simulink model "MinTimeClimbSim"  (R2019a)
settings: Solver=ode1  StartTime=0.0  StopTime=600  FixedStep=tstep  RelTol=1e-3
InitFcn:
  | initSim;
StopFcn:
  | plotSimSolution;
values from neighbouring files (symbols this model uses):
  par = problem.data    [initSim.m]
  tstep = 0.1    [initSim.m]
undefined symbols (not defined in the file or in its folder): F, m, MIL, Moderate, problem
libraries: aerolibwind2 x1, sharedtransform x1
settings Model: Creator=yn15  LastModifiedBy=Yuanb
settings DataIOCC: ReturnWorkspaceOutputs=off
settings OptimizationCC: LifeSpan=inf
settings DebuggingCC: SFUnexpectedBacktrackingDiag=warning  SFNoUnconditionalDefaultTransitionDiag=warning  SFExecutionAtInitializationDiag=none  ArithmeticOperatorsInVariantConditions=warning
settings SFSimCC: SimUseLocalCustomCode=off
settings RTWCC: RTWUseLocalCustomCode=off
settings CodeAppCC: StateflowObjectComments=on
settings GRTTargetCC: TargetLangStandard=C89/C90 (ANSI)
settings ConfigComp: CovMetricSettings=dw  CovHtmlReporting=on  CovSaveCumulativeToWorkspaceVar=on  CovSaveSingleToWorkspaceVar=on  CovExternalEMLEnable=off

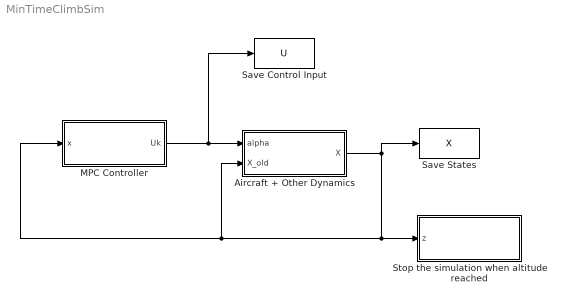
== system MinTimeClimbSim ==
  Aircraft + Other Dynamics : Subsystem
  "MPC Controller " : Subsystem
  Save Control Input : ToWorkspace  VariableName=U  SampleTime=-1
      settings: Save2DSignal=2-D array (concatenate along first dimension)
  Save States : ToWorkspace  VariableName=X  SampleTime=-1
  "Stop the simulation when altitude reached " : Subsystem
  wires:
  "MPC Controller "/1(Uk) -> Aircraft + Other Dynamics/1(alpha), Save Control Input/1
  Aircraft + Other Dynamics/1(X) -> Save States/1, "Stop the simulation when altitude reached "/1(z), Aircraft + Other Dynamics/2("X_old "), "MPC Controller "/1(x)

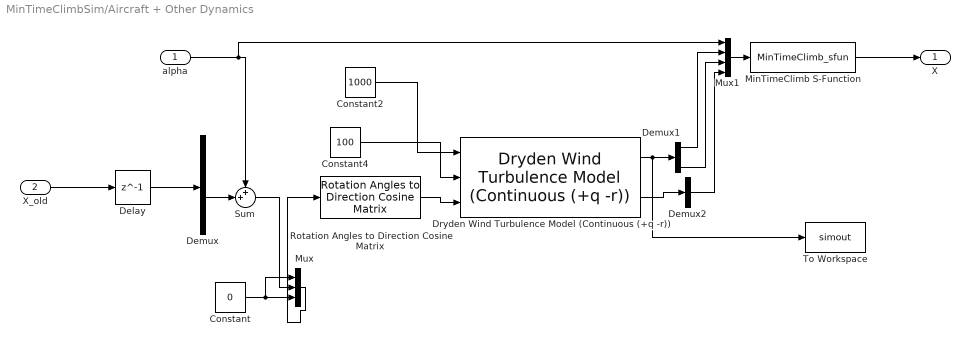
== system MinTimeClimbSim/Aircraft + Other Dynamics ==
  alpha : Inport
  "X_old " : Inport  Port=2
  Constant : Constant  Value=0  SampleTime=-1
  Constant2 : Constant  Value=1000  SampleTime=-1
  Constant4 : Constant  Value=100  SampleTime=-1
  Delay : Delay  DelayLength=1  InitialCondition=[problem.states.x0]
  Demux : Demux
  Demux1 : Demux  Outputs=3
  Demux2 : Demux  Outputs=3
  Dryden Wind Turbulence Model (Continuous (+q -r)) : aerolibwind2/Dryden Wind Turbulence Model  (Continuous (+q -r))  units=Metric (MKS)  spec=MIL-F-8785C  model=Continuous Dryden (+q -r)  W20=15  Wdeg=0  TurbProb=10^-3 - Moderate  L_high=533.4  Wingspan=10  ts=tstep  Seed=[23341 23342 23343 23344]  T_on=on
      settings: SourceProductName=Aerospace Blockset
  MinTimeClimb S-Function : S-Function  FunctionName=MinTimeClimb_sfun  Parameters=par;problem.states.x0  SFunctionDeploymentMode=off  EnableBusSupport=off
  Mux : Mux  Inputs=3
  Mux1 : Mux
  Rotation Angles to Direction Cosine Matrix : sharedtransform/Rotation Angles to Direction Cosine Matrix  rotationOrder=ZYX  aMode=aMode
      settings: SourceProductBaseCode=AE
  Sum : Sum  Inputs=++|
  To Workspace : ToWorkspace  VariableName=simout  SaveFormat=Structure With Time  SampleTime=-1
  X : Outport
  wires:
  alpha/1 -> Mux1/1, Sum/1
  MinTimeClimb S-Function/1 -> X/1
  "X_old "/1 -> Delay/1
  Demux/3 -> Sum/2
  Mux/1 -> Rotation Angles to Direction Cosine Matrix/1
  Constant/1 -> Mux/3, Mux/1
  Dryden Wind Turbulence Model (Continuous (+q -r))/2 -> Demux2/1
  Sum/1 -> Mux/2
  Mux1/1 -> MinTimeClimb S-Function/1
  Dryden Wind Turbulence Model (Continuous (+q -r))/1 -> To Workspace/1, Demux1/1
  Delay/1 -> Demux/1
  Demux1/1 -> Mux1/2
  Demux1/3 -> Mux1/3
  Demux2/2 -> Mux1/4
  Rotation Angles to Direction Cosine Matrix/1 -> Dryden Wind Turbulence Model (Continuous (+q -r))/3
  Constant2/1 -> Dryden Wind Turbulence Model (Continuous (+q -r))/1
  Constant4/1 -> Dryden Wind Turbulence Model (Continuous (+q -r))/2

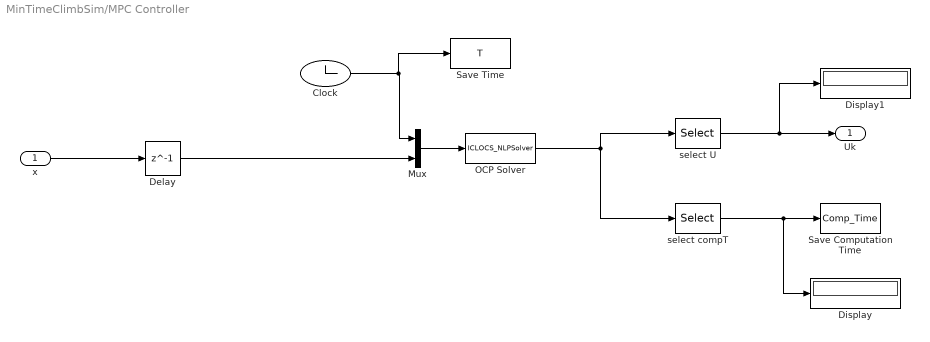
== system MinTimeClimbSim/MPC Controller  ==
  x : Inport
  Clock : Clock
  Delay : Delay  DelayLength=1  InitialCondition=[problem.states.x0]
  Display : Display
  Display1 : Display
  Mux : Mux  Inputs=2
  OCP Solver : MATLABFcn  MATLABFcn=ICLOCS_NLPSolver  OutputDimensions=m+2
  "Save Computation Time " : ToWorkspace  VariableName=Comp_Time  SampleTime=tstep
      settings: Save2DSignal=2-D array (concatenate along first dimension)
  Save Time : ToWorkspace  VariableName=T  SampleTime=-1
      settings: Save2DSignal=2-D array (concatenate along first dimension)
  select U : Selector  IndexOptions=Index vector (dialog)  Indices=3:m+2  OutputSizes=1
  select compT : Selector  IndexOptions=Index vector (dialog)  Indices=2  OutputSizes=1
  Uk : Outport
  wires:
  select U/1 -> Display1/1, Uk/1
  x/1 -> Delay/1
  OCP Solver/1 -> select compT/1, select U/1
  Clock/1 -> Save Time/1, Mux/1
  Mux/1 -> OCP Solver/1
  Delay/1 -> Mux/2
  select compT/1 -> Display/1, "Save Computation Time "/1

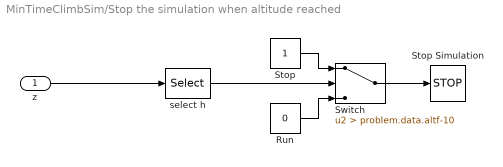
== system MinTimeClimbSim/Stop the simulation when altitude reached  ==
  z : Inport
  Run : Constant  Value=0
  Stop : Constant
  Stop Simulation : Stop
  Switch : Switch  Criteria=u2 > Threshold  Threshold=problem.data.altf-10
  select h : Selector  IndexOptions=Index vector (dialog)  Indices=1  OutputSizes=1
  wires:
  Switch/1 -> Stop Simulation/1
  z/1 -> select h/1
  Stop/1 -> Switch/1
  Run/1 -> Switch/3
  select h/1 -> Switch/2
